simulink library "csu_isb_initialize_state_bus_lib"  (R2014b)
settings: Solver=ode45  StartTime=0.0  StopTime=10.0  RelTol=1e-3
values from neighbouring files (symbols this model uses):
  ini_quaternion_v = compute_scenario_initial_quatnerion(ini_j2000_or_topo, ini_rotx, ini_roty, ini_rotz, ini_epoch_seconds, ini_moon_rotation_rate, ini_Tmat_MCMF_to_Topocentric, ini_hour, ini_minute, ini_seconds, earth_moon_rotation_matrix_select)    [csu_ini_initial_conditions_prep.m]
undefined symbols (not defined in the file or in its folder): ini_position_v, ini_velocity_v
libraries: simulink x3, util_info_lib x1
settings Model: Creator=escrane  LastModifiedBy=mstewart

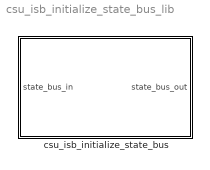
== system csu_isb_initialize_state_bus_lib ==
  csu_isb_initialize_state_bus : Subsystem

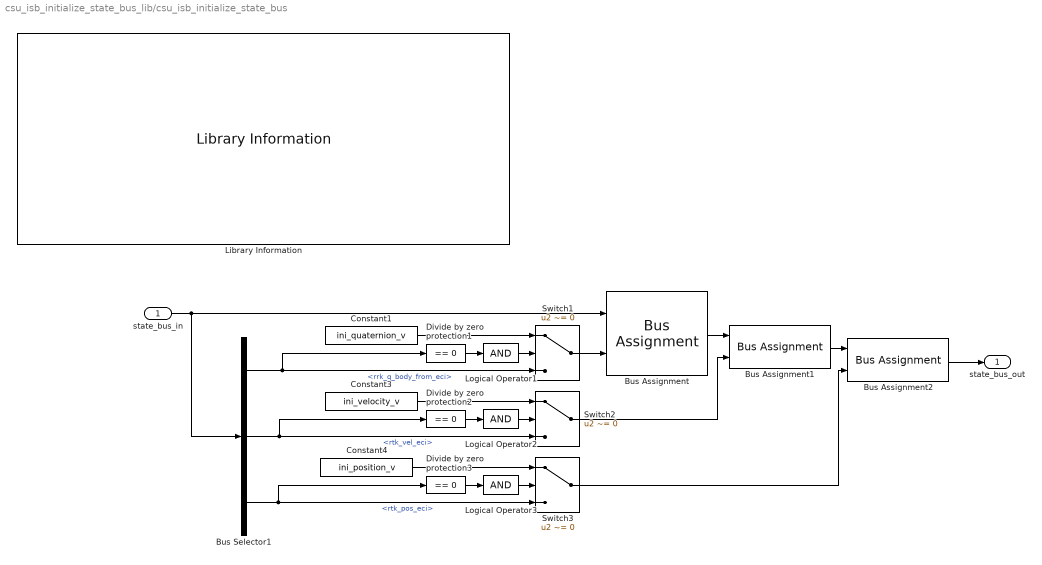
== system csu_isb_initialize_state_bus_lib/csu_isb_initialize_state_bus ==
  state_bus_in : Inport
  Bus Assignment : BusAssignment  AssignedSignals=rrk_q_body_from_eci
  Bus Assignment1 : BusAssignment  AssignedSignals=rtk_vel_eci
  Bus Assignment2 : BusAssignment  AssignedSignals=rtk_pos_eci
  Bus Selector1 : BusSelector  OutputSignals=rrk_q_body_from_eci,rtk_vel_eci,rtk_pos_eci
  Constant1 : Constant  Value=ini_quaternion_v
  Constant3 : Constant  Value=ini_velocity_v
  Constant4 : Constant  Value=ini_position_v
  Divide by zero protection1 : simulink/Logic and Bit Operations/Compare To Constant  relop===  const=0  OutDataTypeStr=uint8
  Divide by zero protection2 : simulink/Logic and Bit Operations/Compare To Constant  relop===  const=0  OutDataTypeStr=uint8
  Divide by zero protection3 : simulink/Logic and Bit Operations/Compare To Constant  relop===  const=0  OutDataTypeStr=uint8
  Library Information : util_info_lib/Library Information  owner='NONE'
  Logical Operator1 : Logic  Inputs=1  AllPortsSameDT=off  OutDataTypeStr=boolean
  Logical Operator2 : Logic  Inputs=1  AllPortsSameDT=off  OutDataTypeStr=boolean
  Logical Operator3 : Logic  Inputs=1  AllPortsSameDT=off  OutDataTypeStr=boolean
  Switch1 : Switch  Criteria=u2 ~= 0
  Switch2 : Switch  Criteria=u2 ~= 0
  Switch3 : Switch  Criteria=u2 ~= 0
  state_bus_out : Outport
  wires:
  Bus Selector1/1 -> Switch1/3, Divide by zero protection1/1  "<rrk_q_body_from_eci>"
  Divide by zero protection1/1 -> Logical Operator1/1
  Logical Operator1/1 -> Switch1/2
  Bus Selector1/2 -> Switch2/3, Divide by zero protection2/1  "<rtk_vel_eci>"
  Divide by zero protection2/1 -> Logical Operator2/1
  Logical Operator2/1 -> Switch2/2
  Constant3/1 -> Switch2/1
  Constant1/1 -> Switch1/1
  Bus Selector1/3 -> Divide by zero protection3/1, Switch3/3  "<rtk_pos_eci>"
  Divide by zero protection3/1 -> Logical Operator3/1
  Logical Operator3/1 -> Switch3/2
  Constant4/1 -> Switch3/1
  Switch1/1 -> Bus Assignment/2
  Bus Assignment/1 -> Bus Assignment1/1
  Switch2/1 -> Bus Assignment1/2
  Bus Assignment1/1 -> Bus Assignment2/1
  Switch3/1 -> Bus Assignment2/2
  Bus Assignment2/1 -> state_bus_out/1
  state_bus_in/1 -> Bus Selector1/1, Bus Assignment/1
